simulink subsystem "Luenberger_Load_Observer"  (R2024a)
settings: Solver=VariableStepAuto  StartTime=0.0  StopTime=10.0  RelTol=1e-3
undefined symbols (not defined in the file or in its folder): DiscIntNeverNeededParam, Ltau, motor
settings Model: Creator=rdelpoux  LastModifiedBy=rdelpoux

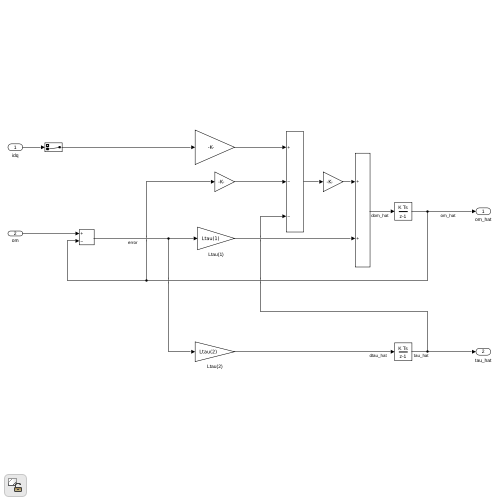
[thumbnail: Simulink's stored preview of the top-level diagram]
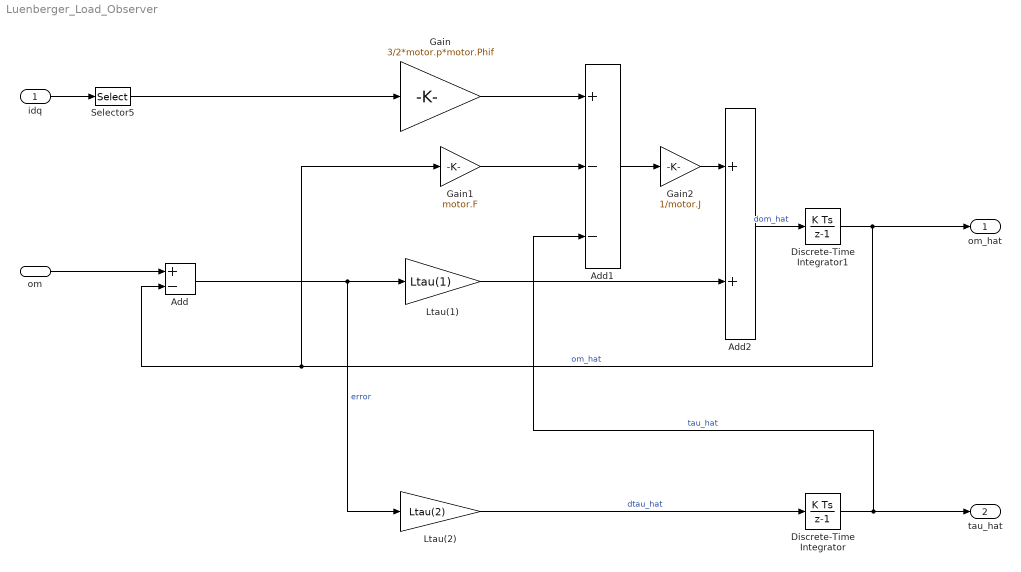
== system Luenberger_Load_Observer ==
  idq : Inport
  om : Inport  Port=2
  Add : Sum  Inputs=+-
  Add1 : Sum  Inputs=+--
  Add2 : Sum
  Discrete-Time Integrator : DiscreteIntegrator  SampleTime=1e-4  OutDataTypeStr=single  ICPrevOutput=DiscIntNeverNeededParam  ICPrevScaledInput=DiscIntNeverNeededParam
  Discrete-Time Integrator1 : DiscreteIntegrator  SampleTime=1e-4  OutDataTypeStr=single  ICPrevOutput=DiscIntNeverNeededParam  ICPrevScaledInput=DiscIntNeverNeededParam
  Gain : Gain  Gain=3/2*motor.p*motor.Phif
  Gain1 : Gain  Gain=motor.F
  Gain2 : Gain  Gain=1/motor.J
  Ltau(1) : Gain  Gain=Ltau(1)
  Ltau(2) : Gain  Gain=Ltau(2)
  Selector5 : Selector  InputPortWidth=2  IndexOptions=Index vector (dialog)  Indices=[2]  OutputSizes=1
  om_hat : Outport
  tau_hat : Outport  Port=2
  wires:
  idq/1 -> Selector5/1
  Ltau(1)/1 -> Add2/2
  Add2/1 -> Discrete-Time Integrator1/1  "dom_hat"
  Add1/1 -> Gain2/1
  om/1 -> Add/1
  Discrete-Time Integrator/1 -> Add1/3, tau_hat/1  "tau_hat"
  Gain2/1 -> Add2/1
  Add/1 -> Ltau(1)/1, Ltau(2)/1  "error"
  Discrete-Time Integrator1/1 -> Add/2, Gain1/1, om_hat/1  "om_hat"
  Gain/1 -> Add1/1
  Gain1/1 -> Add1/2
  Ltau(2)/1 -> Discrete-Time Integrator/1  "dtau_hat"
  Selector5/1 -> Gain/1
